simulink model "Courant_BO"  (R2024b)
settings: Solver=VariableStepAuto  StartTime=0.0  StopTime=2  RelTol=1e-3
values from neighbouring files (symbols this model uses):
  Cfs = 0.0328    [parametres.m]
  f = 0.0006    [parametres.m]
  Jm = 79e-3*1e-4    (= 7.9e-06)    [parametres.m]
  Jv = 10.8*Lv*1e-6    (= 3.24e-06)    [parametres.m]
  K_codeur = 8192/360    (= 22.7555555556)    [parametres.m]
  K_meca = 1/110    (= 0.00909090909091)    [parametres.m]
  Kc = 29.2e-3    (= 0.0292)    [parametres.m]
  Ke = 1/Ke    (= 0.0291137091022)    [parametres.m]
  KI_i = 200    [parametres.m]
  KP_i = 800    [parametres.m]
  Lm = 0.191e-3    (= 0.000191)    [parametres.m]
  Rm = 0.582    [parametres.m]
  Umax = 24    [parametres.m]
settings Model: Creator=xpess  LastModifiedBy=xpess
settings RTWCC: GPUComputeCapability=3.5

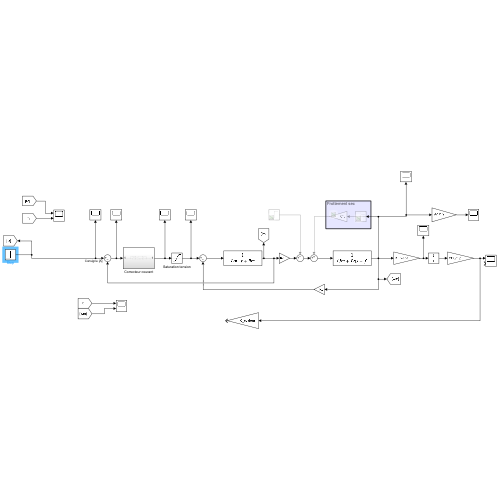
[thumbnail: Simulink's stored preview of the top-level diagram]
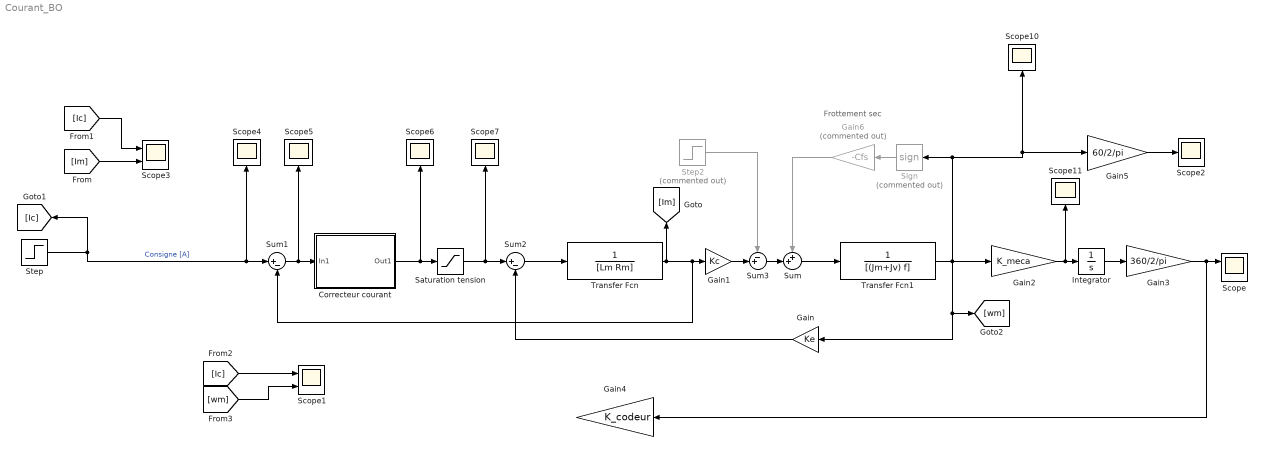
== system Courant_BO ==
  note: Frottement sec
  Correcteur courant : Subsystem
  Gain : Gain  Gain=Ke
  Gain1 : Gain  Gain=Kc
  Gain2 : Gain  Gain=K_meca
  Gain3 : Gain  Gain=360/2/pi
  Gain4 : Gain  Gain=K_codeur
  Gain5 : Gain  Gain=60/2/pi
  Gain6 : Gain  Commented=on  Gain=-Cfs
  Integrator : Integrator
  Saturation tension : Saturate  UpperLimit=Umax  LowerLimit=-Umax
  Scope : Scope  NumInputPorts=2
  Scope1 : Scope  NumInputPorts=2
  Scope{2,4..7,10..11} (7 alike) : Scope
  Scope3 : Scope  NumInputPorts=2
  Sign : Signum  Commented=on  ZeroCross=off
  Step : Step  Time=0.03  After=2  SampleTime=0
  Step2 : Step  Commented=on  After=0  SampleTime=0
  Sum : Sum  Inputs=++|
  Sum1 : Sum  Inputs=|+-
  Sum2 : Sum  Inputs=|+-
  Sum3 : Sum  Inputs=-+|
  Transfer Fcn : TransferFcn  Denominator=[Lm Rm]
  Transfer Fcn1 : TransferFcn  Denominator=[(Jm+Jv) f]
  wires:
  Transfer Fcn/1 -> Gain1/1, Sum1/2, [Im]
  Gain2/1 -> Scope11/1, Integrator/1
  Gain3/1 -> Scope/1, Gain4/1
  Step/1 -> Scope4/1, Sum1/1, [Ic]  "Consigne [A]"
  Gain1/1 -> Sum3/2
  Integrator/1 -> Gain3/1
  Gain/1 -> Sum2/2
  Sum1/1 -> Scope5/1, Correcteur courant/1(In1)
  Correcteur courant/1(Out1) -> Scope6/1, Saturation tension/1
  Sum2/1 -> Transfer Fcn/1
  Saturation tension/1 -> Sum2/1, Scope7/1
  Gain6/1 -> Sum/1
  Transfer Fcn1/1 -> Scope10/1, Gain5/1, Sign/1, Gain2/1, [wm], Gain/1
  Sign/1 -> Gain6/1
  Sum3/1 -> Sum/2
  Step2/1 -> Sum3/1
  Sum/1 -> Transfer Fcn1/1
  Gain5/1 -> Scope2/1
  [Im] -> Scope3/2
  [Ic] -> Scope3/1
  [Ic] -> Scope1/1
  [wm] -> Scope1/2

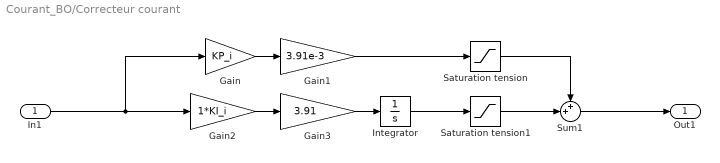
== system Courant_BO/Correcteur courant ==
  In1 : Inport
  Gain : Gain  Gain=KP_i
  Gain1 : Gain  Gain=3.91e-3
  Gain2 : Gain  Gain=1*KI_i
  Gain3 : Gain  Gain=3.91
  Integrator : Integrator
  Saturation tension : Saturate  UpperLimit=Umax*10  LowerLimit=-Umax*10
  Saturation tension1 : Saturate  UpperLimit=Umax*10  LowerLimit=-Umax*10
  Sum1 : Sum  Inputs=++|
  Out1 : Outport
  wires:
  Sum1/1 -> Out1/1
  Gain3/1 -> Integrator/1
  Integrator/1 -> Saturation tension1/1
  Gain2/1 -> Gain3/1
  In1/1 -> Gain2/1, Gain/1
  Gain/1 -> Gain1/1
  Gain1/1 -> Saturation tension/1
  Saturation tension/1 -> Sum1/1
  Saturation tension1/1 -> Sum1/2
